simulink library "acc"  (R2021b)
settings: Solver=VariableStepAuto  StartTime=0.0  StopTime=10.0  RelTol=1e-3
undefined symbols (not defined in the file or in its folder): AACC_CondensorFanReq_X_enum, AACC_EWP1CCUReq_X_C, AACC_EWP1EDUReq_X_C, AACC_EWP1HVBReq_X_C, AACC_EWP2CCUReq_X_C, AACC_EWP2EDUReq_X_C, AACC_EWP2HVBReq_X_C, AACC_FWV1CCUReq_X_C, AACC_FWV1EDUReq_X_C, AACC_FWV1HVBReq_X_C, AACC_FWV2CCUReq_X_C, AACC_FWV2EDUReq_X_C, AACC_FWV2HVBReq_X_C, AACC_TWVCCUReq_X_C, AACC_TWVEDUReq_X_C, AACC_TWVHVBReq_X_C, ENUM_ACCMODE_CHARGING, ENUM_ACCMODE_COOLING, ENUM_ACCMODE_OFF, ENUM_ACCMODE_SERVICE, ENUM_ACREQ_COOLING, ENUM_ACREQ_NOREQUEST, ENUM_CHILLERINITREQ_NONE, ENUM_CHILLERINITREQ_START, ENUM_CHILLERINITREQ_WAITING, ENUM_CHILLERINITSTA_FINISH, ENUM_CHILLERINITSTA_INPROCESS, ENUM_COOLFANREQ_HI, ENUM_COOLFANREQ_LOW, ENUM_COOLFANREQ_OFF, ENUM_LVBATTSTA_FAIL, ENUM_LVBATTSTA_NORMAL, ENUM_PMMMODE_CHARGE, ENUM_PMMMODE_DRIVE, ENUM_PMMMODE_LVBATCHRG, ENUM_PMMMODE_POWERUP, ENUM_THCMSYS_INACTIVE, FALSE, KACC_CCUFanHighOffTemp_C, KACC_CCUFanHighOnTemp_C, KACC_CCUFanLowOffTemp_C, KACC_CCUFanLowOnTemp_C, KACC_ChillerInitTime_s, KACC_ChillerStartTime_s, KACC_DCDCCalPwrAvailRsv_kW, KACC_EDUFanHighOffTemp_C, KACC_EDUFanHighOnTemp_C, KACC_EDUFanLowOffTemp_C, KACC_EDUFanLowOnTemp_C, KACC_EWP1CalDutyVal_pct, KACC_EWP1CalON_flg, KACC_EWP2CalDutyVal_pct, KACC_EWP2CalON_flg, KACC_EXVCalON_flg, KACC_EXVCalVal_cnt, KACC_FanCalON_flg, KACC_FanCalVal_enum, KACC_FWV1CalON_flg, KACC_FWV1CalVal_flg, KACC_FWV2CalON_flg ... (+51)
libraries: simulink x1
(part 2 of 2)

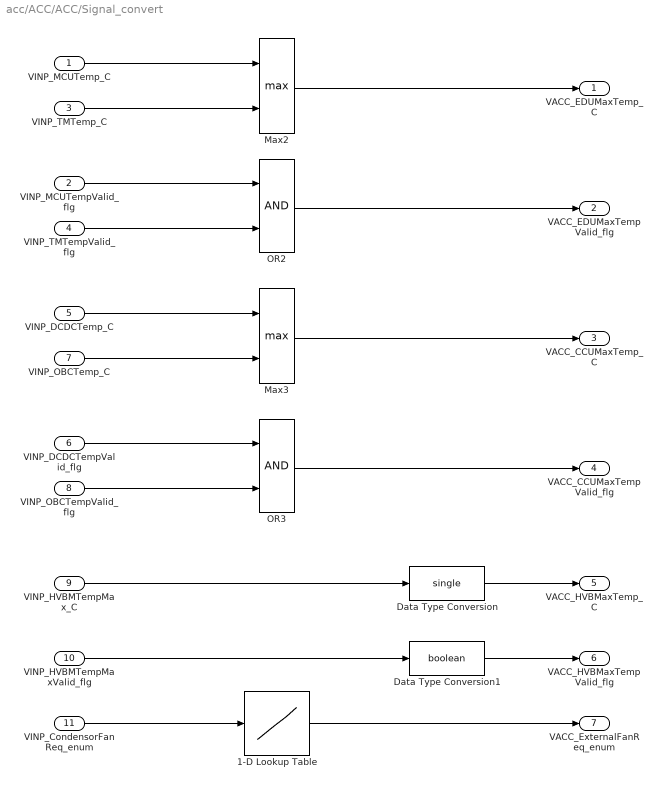
== system acc/ACC/ACC/Signal_convert ==
  VINP_MCUTemp_C : Inport
  VINP_MCUTempValid_flg : Inport  Port=2
  VINP_TMTemp_C : Inport  Port=3
  VINP_TMTempValid_flg : Inport  Port=4
  VINP_DCDCTemp_C : Inport  Port=5
  VINP_DCDCTempValid_flg : Inport  Port=6
  VINP_OBCTemp_C : Inport  Port=7
  VINP_OBCTempValid_flg : Inport  Port=8
  VINP_HVBMTempMax_C : Inport  Port=9
  VINP_HVBMTempMaxValid_flg : Inport  Port=10
  VINP_CondensorFanReq_enum : Inport  Port=11
  1-D Lookup Table : Lookup_n-D  NumberOfTableDimensions=1  BreakpointsForDimension1=AACC_CondensorFanReq_X_enum  Table=MACC_CondensorFanReq_Y_enum  InterpMethod=Flat  InternalRulePriority=Speed  RndMeth=Simplest  InputSameDT=on
  Data Type Conversion : DataTypeConversion  OutDataTypeStr=single
  Data Type Conversion1 : DataTypeConversion  OutDataTypeStr=boolean
  Max2 : MinMax  Function=max  Inputs=2
  Max3 : MinMax  Function=max  Inputs=2
  OR2 : Logic  AllPortsSameDT=off  OutDataTypeStr=boolean
  OR3 : Logic  AllPortsSameDT=off  OutDataTypeStr=boolean
  VACC_EDUMaxTemp_C : Outport
  VACC_EDUMaxTempValid_flg : Outport  Port=2
  VACC_CCUMaxTemp_C : Outport  Port=3
  VACC_CCUMaxTempValid_flg : Outport  Port=4
  VACC_HVBMaxTemp_C : Outport  Port=5
  VACC_HVBMaxTempValid_flg : Outport  Port=6
  VACC_ExternalFanReq_enum : Outport  Port=7
  wires:
  Data Type Conversion1/1 -> VACC_HVBMaxTempValid_flg/1
  Data Type Conversion/1 -> VACC_HVBMaxTemp_C/1
  1-D Lookup Table/1 -> VACC_ExternalFanReq_enum/1
  VINP_CondensorFanReq_enum/1 -> 1-D Lookup Table/1
  VINP_HVBMTempMaxValid_flg/1 -> Data Type Conversion1/1
  VINP_HVBMTempMax_C/1 -> Data Type Conversion/1
  OR3/1 -> VACC_CCUMaxTempValid_flg/1
  Max3/1 -> VACC_CCUMaxTemp_C/1
  VINP_OBCTempValid_flg/1 -> OR3/2
  VINP_DCDCTempValid_flg/1 -> OR3/1
  VINP_DCDCTemp_C/1 -> Max3/1
  VINP_OBCTemp_C/1 -> Max3/2
  OR2/1 -> VACC_EDUMaxTempValid_flg/1
  VINP_TMTempValid_flg/1 -> OR2/2
  VINP_MCUTempValid_flg/1 -> OR2/1
  Max2/1 -> VACC_EDUMaxTemp_C/1
  VINP_TMTemp_C/1 -> Max2/2
  VINP_MCUTemp_C/1 -> Max2/1

== system acc/ACC/ACC/Thermal_Managemant_Mode_Determination ==
  VPMM_SysPowerMode_enum : Inport
  Constant : Constant  Value=KACC_ServiceModeON_flg
  Cooling Mode : Subsystem
  PECoolingMode : Subsystem
  Service Mode : Subsystem
  Subsystem : Subsystem
  VACC_PECoolingMode_enum : Outport  VectorParamsAs1DForOutWhenUnconnected=off
  wires:
  Constant/1 -> Service Mode/1(KACC_ServiceModeON_flg)
  [VACC_CoolingMode_flg] -> PECoolingMode/3(VACC_CoolingMode_flg)
  [VACC_ChargingMode_flg] -> PECoolingMode/2(VACC_ChargingMode_flg)
  [VACC_ServiceMode_flg] -> PECoolingMode/1(VACC_ServiceMode_flg)
  [VPMM_SysPowerMode_enum] -> Subsystem/1(VPMM_SysPowerMode_enum)
  Subsystem/1(VACC_CoolingMode_flg) -> [VACC_CoolingMode_flg]
  PECoolingMode/1(VACC_PECoolingMode_enum) -> VACC_PECoolingMode_enum/1
  [VPMM_SysPowerMode_enum] -> Cooling Mode/1(VPMM_SysPowerMode_enum)
  VPMM_SysPowerMode_enum/1 -> [VPMM_SysPowerMode_enum]
  Service Mode/1(VACC_ServiceMode_flg) -> [VACC_ServiceMode_flg]
  Cooling Mode/1(VACC_ChargingMode_flg) -> [VACC_ChargingMode_flg]

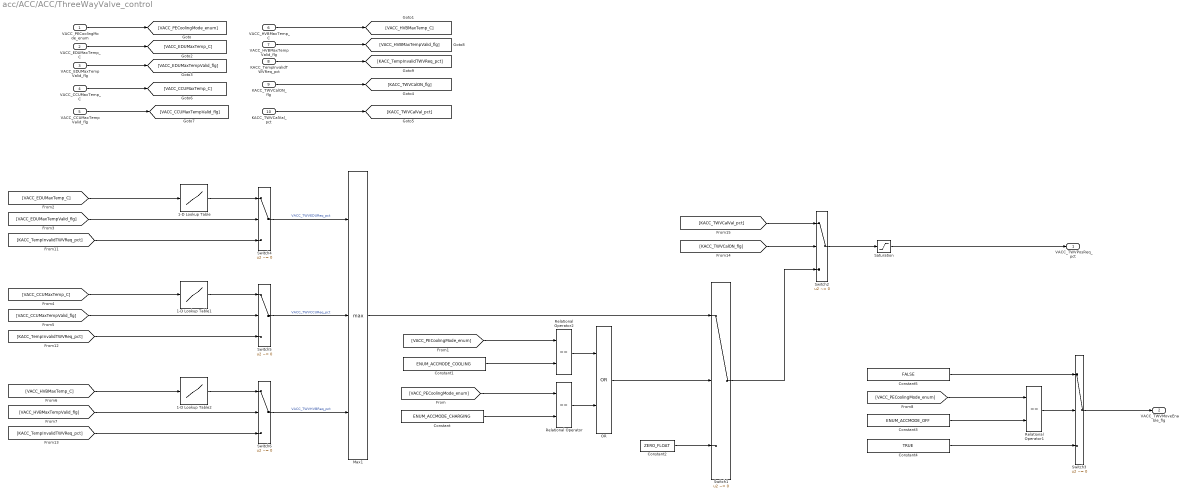
== system acc/ACC/ACC/ThreeWayValve_control ==
  VACC_PECoolingMode_enum : Inport
  VACC_EDUMaxTemp_C : Inport  Port=2
  VACC_EDUMaxTempValid_flg : Inport  Port=3
  VACC_CCUMaxTemp_C : Inport  Port=4
  VACC_CCUMaxTempValid_flg : Inport  Port=5
  VACC_HVBMaxTemp_C : Inport  Port=6
  VACC_HVBMaxTempValid_flg : Inport  Port=7
  KACC_TempInvalidTWVReq_pct : Inport  Port=8
  KACC_TWVCalON_flg : Inport  Port=9
  KACC_TWVCalVal_pct : Inport  Port=10
  1-D Lookup Table : Lookup_n-D  NumberOfTableDimensions=1  BreakpointsForDimension1=AACC_TWVEDUReq_X_C  Table=MACC_TWVEDUReq_Y_pct  UseLastTableValue=on  InternalRulePriority=Speed  RndMeth=Simplest  InputSameDT=on
  1-D Lookup Table1 : Lookup_n-D  NumberOfTableDimensions=1  BreakpointsForDimension1=AACC_TWVCCUReq_X_C  Table=MACC_TWVCCUReq_Y_pct  UseLastTableValue=on  InternalRulePriority=Speed  RndMeth=Simplest  InputSameDT=on
  1-D Lookup Table2 : Lookup_n-D  NumberOfTableDimensions=1  BreakpointsForDimension1=AACC_TWVHVBReq_X_C  Table=MACC_TWVHVBReq_Y_pct  UseLastTableValue=on  InternalRulePriority=Speed  RndMeth=Simplest  InputSameDT=on
  Constant : Constant  Value=ENUM_ACCMODE_CHARGING
  Constant1 : Constant  Value=ENUM_ACCMODE_COOLING
  Constant2 : Constant  Value=ZERO_FLOAT
  Constant3 : Constant  Value=ENUM_ACCMODE_OFF
  Constant4 : Constant  Value=TRUE
  Constant5 : Constant  Value=FALSE
  Max1 : MinMax  Function=max  Inputs=3
  OR : Logic  Operator=OR  AllPortsSameDT=off  OutDataTypeStr=boolean
  Relational Operator : RelationalOperator  Operator===  OutDataTypeStr=boolean  RndMeth=Simplest
  Relational Operator1 : RelationalOperator  Operator===  OutDataTypeStr=boolean  RndMeth=Simplest
  Relational Operator2 : RelationalOperator  Operator===  OutDataTypeStr=boolean  RndMeth=Simplest
  Saturation : Saturate  UpperLimit=100  LowerLimit=0
      settings: AttributesFormatString=|
      | LowerLimi: %<LowerLimit>
      | UpperLimit: %<UpperLimit>
  Switch{1..6} (6 alike) : Switch  Criteria=u2 ~= 0
      settings: AttributesFormatString=%<Criteria>
  VACC_TWVPosReq_pct : Outport
  VACC_TWVMoveEnable_flg : Outport  Port=2
  wires:
  Constant4/1 -> Switch3/3
  Constant5/1 -> Switch3/1
  Switch3/1 -> VACC_TWVMoveEnable_flg/1
  Relational Operator1/1 -> Switch3/2
  [VACC_PECoolingMode_enum] -> Relational Operator1/1
  Constant3/1 -> Relational Operator1/2
  Switch5/1 -> Max1/2  "VACC_TWVCCUReq_pct"
  Switch4/1 -> Max1/1  "VACC_TWVEDUReq_pct"
  KACC_TempInvalidTWVReq_pct/1 -> [KACC_TempInvalidTWVReq_pct]
  VACC_HVBMaxTempValid_flg/1 -> [VACC_HVBMaxTempValid_flg]
  VACC_CCUMaxTempValid_flg/1 -> [VACC_CCUMaxTempValid_flg]
  VACC_CCUMaxTemp_C/1 -> [VACC_CCUMaxTemp_C]
  VACC_EDUMaxTempValid_flg/1 -> [VACC_EDUMaxTempValid_flg]
  VACC_EDUMaxTemp_C/1 -> [VACC_EDUMaxTemp_C]
  Constant2/1 -> Switch1/3
  OR/1 -> Switch1/2
  Relational Operator/1 -> OR/2
  Relational Operator2/1 -> OR/1
  VACC_HVBMaxTemp_C/1 -> [VACC_HVBMaxTemp_C]
  Switch1/1 -> Switch2/3
  Constant/1 -> Relational Operator/2
  Constant1/1 -> Relational Operator2/2
  Max1/1 -> Switch1/1
  [VACC_PECoolingMode_enum] -> Relational Operator2/1
  [VACC_PECoolingMode_enum] -> Relational Operator/1
  VACC_PECoolingMode_enum/1 -> [VACC_PECoolingMode_enum]
  Switch2/1 -> Saturation/1
  Saturation/1 -> VACC_TWVPosReq_pct/1
  KACC_TWVCalON_flg/1 -> [KACC_TWVCalON_flg]
  KACC_TWVCalVal_pct/1 -> [KACC_TWVCalVal_pct]
  [VACC_EDUMaxTempValid_flg] -> Switch4/2
  [KACC_TempInvalidTWVReq_pct] -> Switch4/3
  [VACC_EDUMaxTemp_C] -> 1-D Lookup Table/1
  1-D Lookup Table/1 -> Switch4/1
  [VACC_CCUMaxTemp_C] -> 1-D Lookup Table1/1
  1-D Lookup Table1/1 -> Switch5/1
  [VACC_CCUMaxTempValid_flg] -> Switch5/2
  [KACC_TempInvalidTWVReq_pct] -> Switch5/3
  Switch6/1 -> Max1/3  "VACC_TWVHVBReq_pct"
  1-D Lookup Table2/1 -> Switch6/1
  [VACC_HVBMaxTempValid_flg] -> Switch6/2
  [VACC_HVBMaxTemp_C] -> 1-D Lookup Table2/1
  [KACC_TempInvalidTWVReq_pct] -> Switch6/3
  [KACC_TWVCalON_flg] -> Switch2/2
  [KACC_TWVCalVal_pct] -> Switch2/1

== system acc/ACC/THCM/THCM_Available_Check ==
  VPMM_HVPwrSta_flg : Inport
  Constant4 : Constant  Value=ENUM_THCMSYS_INACTIVE
  Constant5 : Constant  Value=KACC_HVTHCMSysAvail_enum_ovrdflg
  Constant6 : Constant  Value=KACC_HVTHCMSysAvail_enum_ovrdval
  Constant7 : Constant  Value=ENUM_THCMSYS_INACTIVE
  Switch2 : Switch  Criteria=u2 ~= 0
      settings: AttributesFormatString=<%<Criteria>>
  Switch3 : Switch  Criteria=u2 ~= 0
      settings: AttributesFormatString=<%<Criteria>>
  VACC_HVTHCMSysAvail_enum : Outport
  wires:
  Constant5/1 -> Switch3/2
  Constant4/1 -> Switch2/3
  Switch2/1 -> VACC_HVTHCMSysAvail_enum/1  "VACC_HVTHCMSysAvail_enum"
  Switch3/1 -> Switch2/1
  VPMM_HVPwrSta_flg/1 -> Switch2/2
  Constant6/1 -> Switch3/1
  Constant7/1 -> Switch3/3

== system acc/ACC/THCM/THCM_Available_Power ==
  VPMM_HVPwrSta_flg : Inport
  VINP_HVBPwrAvailDchrg_kW : Inport  Port=2
  VINP_FrMCUDCBusVolt_V : Inport  Port=3
  VINP_FrMCUDCBusCurr_A : Inport  Port=4
  VINP_RrMCUDCBusVolt_V : Inport  Port=5
  VINP_RrMCUDCBusCurr_A : Inport  Port=6
  Add : Sum
  Add1 : Sum  Inputs=+-
  Constant10 : Constant  Value=KACC_HVPwrAvail4THCM_W_ovrdval
  Constant8 : Constant  Value=ZERO_FLOAT
  Constant9 : Constant  Value=KACC_HVPwrAvail4THCM_W_ovrdflg
  Product : Product
  Product1 : Product
  Saturation : Saturate  UpperLimit=KACC_THCMMaxPwrAvail_W  LowerLimit=0
      settings: AttributesFormatString=|
      | Upper Limit: %<UpperLimit>
      | Lower Limit: %<LowerLimit>
  Switch1 : Switch  Criteria=u2 ~= 0
      settings: AttributesFormatString=<%<Criteria>>
  Switch4 : Switch  Criteria=u2 ~= 0
      settings: AttributesFormatString=<%<Criteria>>
  VACC_VehHVPwrAvail4THCM_W : Outport
  wires:
  Constant10/1 -> Switch4/1
  Switch4/1 -> Switch1/1
  Saturation/1 -> Switch4/3
  Constant8/1 -> Switch1/3
  VPMM_HVPwrSta_flg/1 -> Switch1/2
  Switch1/1 -> VACC_VehHVPwrAvail4THCM_W/1  "VACC_VehHVPwrAvail4THCM_W"
  Constant9/1 -> Switch4/2
  VINP_RrMCUDCBusCurr_A/1 -> Product/2
  VINP_RrMCUDCBusVolt_V/1 -> Product/1
  VINP_FrMCUDCBusCurr_A/1 -> Product1/2
  VINP_FrMCUDCBusVolt_V/1 -> Product1/1
  Product1/1 -> Add/1
  Product/1 -> Add/2
  VINP_HVBPwrAvailDchrg_kW/1 -> Add1/1
  Add/1 -> Add1/2
  Add1/1 -> Saturation/1

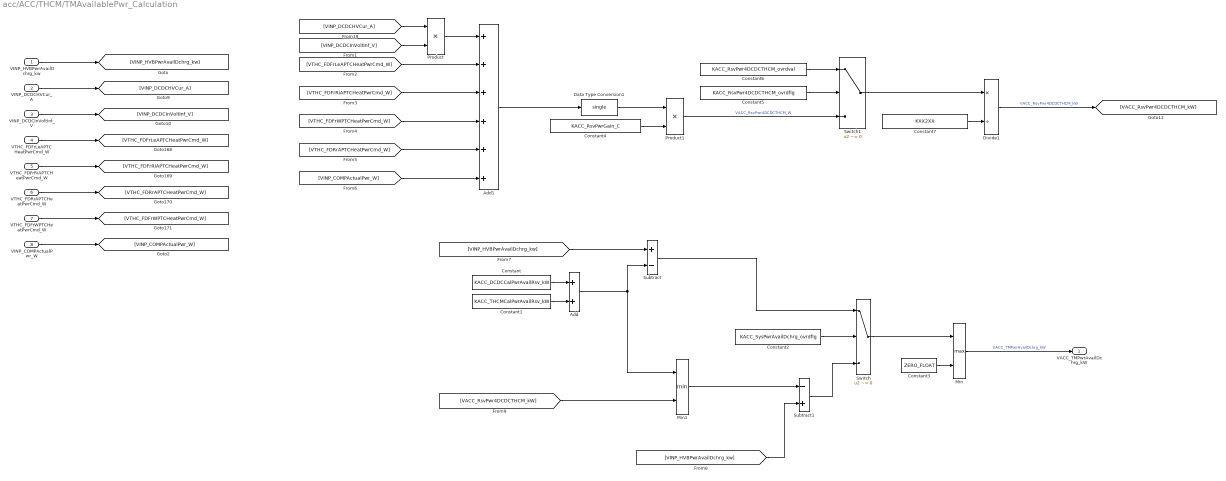
== system acc/ACC/THCM/TMAvailablePwr_Calculation ==
  VINP_HVBPwrAvailDchrg_kw : Inport
  VINP_DCDCHVCur_A : Inport  Port=2
  VINP_DCDCInVoltInf_V : Inport  Port=3
  VTHC_FDFrLeAPTCHeatPwrCmd_W : Inport  Port=4
  VTHC_FDFrRiAPTCHeatPwrCmd_W : Inport  Port=5
  VTHC_FDRrAPTCHeatPwrCmd_W : Inport  Port=6
  VTHC_FDFrWPTCHeatPwrCmd_W : Inport  Port=7
  VINP_COMPActualPwr_W : Inport  Port=8
  Add : Sum
  Add1 : Sum  Inputs=++++++
  Constant : Constant  Value=KACC_DCDCCalPwrAvailRsv_kW
  Constant1 : Constant  Value=KACC_THCMCalPwrAvailRsv_kW
  Constant2 : Constant  Value=KACC_SysPwrAvailDchrg_ovrdflg
  Constant3 : Constant  Value=ZERO_FLOAT
  Constant4 : Constant  Value=KACC_RsvPwrGain_C
  Constant5 : Constant  Value=KACC_RsvPwr4DCDCTHCM_ovrdflg
  Constant6 : Constant  Value=KACC_RsvPwr4DCDCTHCM_ovrdval
  Constant7 : Constant  Value=KXX2XX
  Data Type Conversion1 : DataTypeConversion  OutDataTypeStr=single
  Divide1 : Product  Inputs=*/
  Min : MinMax  Function=max  Inputs=2
  Min1 : MinMax  Inputs=2
  Product : Product
  Product1 : Product
  Subtract : Sum  Inputs=+-
  Subtract1 : Sum  Inputs=-+
  Switch : Switch  Criteria=u2 ~= 0
      settings: AttributesFormatString=<%<Criteria>>
  Switch1 : Switch  Criteria=u2 ~= 0
  VACC_TMPwrAvailDchrg_kW : Outport
  wires:
  Min1/1 -> Subtract1/1
  [VINP_HVBPwrAvailDchrg_kw] -> Subtract1/2
  [VINP_HVBPwrAvailDchrg_kw] -> Subtract/1
  Subtract1/1 -> Switch/3
  [VACC_RsvPwr4DCDCTHCM_kW] -> Min1/2
  Data Type Conversion1/1 -> Product1/1
  Constant5/1 -> Switch1/2
  Add1/1 -> Data Type Conversion1/1
  Switch1/1 -> Divide1/1
  Divide1/1 -> [VACC_RsvPwr4DCDCTHCM_kW]  "VACC_RsvPwr4DCDCTHCM_kW"
  [VINP_DCDCInVoltInf_V] -> Product/2
  [VINP_DCDCHVCur_A] -> Product/1
  Product/1 -> Add1/1
  [VTHC_FDRrAPTCHeatPwrCmd_W] -> Add1/5
  Constant6/1 -> Switch1/1
  Constant4/1 -> Product1/2
  [VTHC_FDFrRiAPTCHeatPwrCmd_W] -> Add1/3
  Product1/1 -> Switch1/3  "VACC_RsvPwr4DCDCTHCM_W"
  [VINP_COMPActualPwr_W] -> Add1/6
  [VTHC_FDFrLeAPTCHeatPwrCmd_W] -> Add1/2
  [VTHC_FDFrWPTCHeatPwrCmd_W] -> Add1/4
  Constant7/1 -> Divide1/2
  VINP_COMPActualPwr_W/1 -> [VINP_COMPActualPwr_W]
  VTHC_FDFrWPTCHeatPwrCmd_W/1 -> [VTHC_FDFrWPTCHeatPwrCmd_W]
  VTHC_FDRrAPTCHeatPwrCmd_W/1 -> [VTHC_FDRrAPTCHeatPwrCmd_W]
  VTHC_FDFrRiAPTCHeatPwrCmd_W/1 -> [VTHC_FDFrRiAPTCHeatPwrCmd_W]
  VTHC_FDFrLeAPTCHeatPwrCmd_W/1 -> [VTHC_FDFrLeAPTCHeatPwrCmd_W]
  VINP_DCDCInVoltInf_V/1 -> [VINP_DCDCInVoltInf_V]
  VINP_DCDCHVCur_A/1 -> [VINP_DCDCHVCur_A]
  Constant/1 -> Add/1
  Constant1/1 -> Add/2
  VINP_HVBPwrAvailDchrg_kw/1 -> [VINP_HVBPwrAvailDchrg_kw]
  Add/1 -> Subtract/2, Min1/1
  Subtract/1 -> Switch/1
  Constant2/1 -> Switch/2
  Switch/1 -> Min/1
  Min/1 -> VACC_TMPwrAvailDchrg_kW/1  "VACC_TMPwrAvailDchrg_kW"
  Constant3/1 -> Min/2

== system acc/ACC/ACC/Thermal_Managemant_Mode_Determination/Cooling Mode ==
  VPMM_SysPowerMode_enum : Inport
  Constant2 : Constant  Value=ENUM_PMMMODE_LVBATCHRG  SampleTime=-1
  Constant4 : Constant  Value=ENUM_PMMMODE_CHARGE  SampleTime=-1
  Logical Operator : Logic  Operator=OR  AllPortsSameDT=off  OutDataTypeStr=boolean
  Relational Operator1 : RelationalOperator  Operator===  OutDataTypeStr=boolean  RndMeth=Nearest
  Relational Operator3 : RelationalOperator  Operator===  OutDataTypeStr=boolean  RndMeth=Nearest
  VACC_ChargingMode_flg : Outport  VectorParamsAs1DForOutWhenUnconnected=off
  wires:
  [VPMM_SysPowerMode_enum] -> Relational Operator3/1
  Constant2/1 -> Relational Operator3/2
  VPMM_SysPowerMode_enum/1 -> [VPMM_SysPowerMode_enum]
  [VPMM_SysPowerMode_enum] -> Relational Operator1/1
  Constant4/1 -> Relational Operator1/2
  Relational Operator3/1 -> Logical Operator/1
  Relational Operator1/1 -> Logical Operator/2
  Logical Operator/1 -> VACC_ChargingMode_flg/1  "VACC_ChargingMode_flg"

== system acc/ACC/ACC/Thermal_Managemant_Mode_Determination/PECoolingMode ==
  VACC_ServiceMode_flg : Inport
  VACC_ChargingMode_flg : Inport  Port=2
  VACC_CoolingMode_flg : Inport  Port=3
  Constant12 : Constant  Value=ENUM_ACCMODE_COOLING  SampleTime=-1
  Constant15 : Constant  Value=ENUM_ACCMODE_OFF  SampleTime=-1
  Constant2 : Constant  Value=ENUM_ACCMODE_CHARGING  SampleTime=-1
  Constant7 : Constant  Value=ENUM_ACCMODE_SERVICE  SampleTime=-1
  Switch1 : Switch  Criteria=u2 ~= 0
  Switch2 : Switch  Criteria=u2 ~= 0
  Switch4 : Switch  Criteria=u2 ~= 0
  VACC_PECoolingMode_enum : Outport  VectorParamsAs1DForOutWhenUnconnected=off
  wires:
  Constant15/1 -> Switch1/3
  Switch4/1 -> VACC_PECoolingMode_enum/1  "VACC_PECoolingMode_enum"
  VACC_CoolingMode_flg/1 -> Switch1/2
  Constant12/1 -> Switch1/1
  VACC_ServiceMode_flg/1 -> Switch4/2
  Constant7/1 -> Switch4/1
  Switch2/1 -> Switch4/3
  VACC_ChargingMode_flg/1 -> Switch2/2
  Switch1/1 -> Switch2/3
  Constant2/1 -> Switch2/1

== system acc/ACC/ACC/Thermal_Managemant_Mode_Determination/Service Mode ==
  KACC_ServiceModeON_flg : Inport
  VACC_ServiceMode_flg : Outport  VectorParamsAs1DForOutWhenUnconnected=off
  wires:
  KACC_ServiceModeON_flg/1 -> VACC_ServiceMode_flg/1  "VACC_ServiceMode_flg"

== system acc/ACC/ACC/Thermal_Managemant_Mode_Determination/Subsystem ==
  VPMM_SysPowerMode_enum : Inport
  Constant1 : Constant  Value=ENUM_PMMMODE_DRIVE  SampleTime=-1
  Constant2 : Constant  Value=ENUM_PMMMODE_POWERUP  SampleTime=-1
  Logical Operator : Logic  Operator=OR  AllPortsSameDT=off  OutDataTypeStr=boolean
  Relational Operator1 : RelationalOperator  Operator===  OutDataTypeStr=boolean  RndMeth=Nearest
  Relational Operator2 : RelationalOperator  Operator===  OutDataTypeStr=boolean  RndMeth=Nearest
  VACC_CoolingMode_flg : Outport  VectorParamsAs1DForOutWhenUnconnected=off
  wires:
  Logical Operator/1 -> VACC_CoolingMode_flg/1  "VACC_CoolingMode_flg"
  Relational Operator1/1 -> Logical Operator/2
  Relational Operator2/1 -> Logical Operator/1
  VPMM_SysPowerMode_enum/1 -> [VPMM_SysPowerMode_enum]
  [VPMM_SysPowerMode_enum] -> Relational Operator2/1
  [VPMM_SysPowerMode_enum] -> Relational Operator1/1
  Constant1/1 -> Relational Operator1/2
  Constant2/1 -> Relational Operator2/2

== stateflow chart acc/ACC/THCM/LVBattSta_Check ==
  state Check_LV_Batt
    state Check_LVBatt_Low
      en:
      VACC_ChkLVBattLowPass_flg = FALSE;
      (default) -> (junction 148) : {VACC_LVBattChkTime_s = 0;}
      (junction 148) -> (junction 149) [order 1] : [VINP_LVBattDet12V_V > KACC_LVBattErrLoThd_V]
      Check_LVBatt_Low -> (junction 148) [order 1]
      (junction 148) -> (junction 150) [order 2] : {VACC_LVBattChkTime_s += task_time_s;}
      (junction 149) -> (junction 151) : {VACC_ChkLVBattLowPass_flg = TRUE;}
      (junction 151) -> (junction 150)
    state Check_LVBatt_High
      en:
      VACC_ChkLVBattHighPass_flg = FALSE;
      (default) -> (junction 159) : {VACC_LVBattChkTime_s = 0;}
      Check_LVBatt_High -> (junction 159) [order 1]
      (junction 159) -> (junction 160) [order 1] : [VINP_LVBattDet12V_V < KACC_LVBattErrHiThd_V]
      (junction 159) -> (junction 161) [order 2] : {VACC_LVBattChkTime_s += task_time_s;}
      (junction 160) -> (junction 162) : {VACC_ChkLVBattHighPass_flg = TRUE;}
      (junction 162) -> (junction 161)
    state Check_LVBatt_Pass
      en:
      VACC_LVBattVoltSta_enum = ENUM_LVBATTSTA_NORMAL;
    state Check_LVBatt_Fail
      en:
      VACC_LVBattVoltSta_enum = ENUM_LVBATTSTA_FAIL;
    (default) -> (junction 130)
    (junction 182) -> (junction 130)
    (junction 180) -> (junction 182)
    (junction 130) -> (junction 132)
    (junction 132) -> (junction 131) [order 2]
    (junction 131) -> Check_LVBatt_Pass
    (junction 132) -> Check_LVBatt_Low [order 1] : [VPMM_LVPwrSta_flg]
    Check_LVBatt_Low -> (junction 133) [order 2] : [VACC_LVBattChkTime_s > KACC_LVBattErrFailtime_s]
    (junction 133) -> (junction 134)
    Check_LVBatt_Low -> Check_LVBatt_High [order 1] : [VACC_ChkLVBattLowPass_flg]
    Check_LVBatt_High -> (junction 134) [order 2] : [VACC_LVBattChkTime_s > KACC_LVBattErrFailtime_s]
    (junction 134) -> Check_LVBatt_Fail
    Check_LVBatt_High -> Check_LVBatt_Pass [order 1] : [VACC_ChkLVBattHighPass_flg]
    Check_LVBatt_Pass -> (junction 173)
    Check_LVBatt_Fail -> (junction 175)
    (junction 173) -> (junction 180)
    (junction 175) -> (junction 173)
  data: task_time_s input; VPMM_LVPwrSta_flg input; VINP_LVBattDet12V_V input; KACC_LVBattErrLoThd_V input; KACC_LVBattErrHiThd_V input; KACC_LVBattErrFailtime_s input; VACC_LVBattVoltSta_enum output uint8; VACC_ChkLVBattHighPass_flg local boolean; VACC_ChkLVBattLowPass_flg local boolean; VACC_LVBattChkTime_s local single; ENUM_LVBATTSTA_FAIL parameter; ENUM_LVBATTSTA_NORMAL parameter; FALSE parameter; TRUE parameter

== stateflow chart acc/ACC/ACC/Chiller_control/Chiller_Initialize ==
  state MainInitialize
    en:
    VACC_ChillerInitFinish_flg = FALSE;
    VACC_ChillerInitTimeout_flg = FALSE;
    VACC_ChillerInitStart_flg = FALSE;
    VACC_ChillerInitReq_enum = ENUM_CHILLERINITREQ_NONE;
    VACC_ChillerMoveEnable_flg = FALSE;
  state ChillerInitialize
    (default) -> (junction 10) : {
        | VACC_TimeChillerInit_s = 0;
        | }
    ChillerInitialize -> (junction 10) [order 1]
    (junction 10) -> (junction 11) : {
        | VACC_ChillerInitReq_enum = ENUM_CHILLERINITREQ_START;
        | VACC_ChillerMoveEnable_flg = TRUE;
        | }
    (junction 11) -> (junction 13) [order 1] : [VINP_ChillerInitState_enum == ENUM_CHILLERINITSTA_INPROCESS]
    (junction 11) -> (junction 17) [order 2] : {
        | VACC_TimeChillerInit_s  += task_time_s;
        | }
    (junction 13) -> (junction 15) : {
        | VACC_ChillerInitStart_flg = TRUE;
        | }
    (junction 15) -> (junction 17)
  state Timeout
    en:
    VACC_ChillerInitTimeout_flg = TRUE;
    VACC_ChillerMoveEnable_flg = FALSE;
  state ChillerStart
    (default) -> (junction 28) : {
        | VACC_TimeChillerStart_s = 0;
        | }
    ChillerStart -> (junction 28) [order 1]
    (junction 28) -> (junction 29) : {
        | VACC_ChillerInitReq_enum = ENUM_CHILLERINITREQ_WAITING;
        | }
    (junction 29) -> (junction 30) [order 1] : [VINP_ChillerInitState_enum == ENUM_CHILLERINITSTA_FINISH]
    (junction 29) -> (junction 31) [order 2] : {
        | VACC_TimeChillerStart_s += task_time_s;
        | }
    (junction 30) -> (junction 32) : {
        | VACC_ChillerInitFinish_flg = TRUE;
        | VACC_ChillerInitReq_enum = ENUM_CHILLERINITREQ_NONE;
        | }
    (junction 32) -> (junction 31)
  (default) -> MainInitialize
  MainInitialize -> ChillerInitialize : [VACC_PECoolingMode_enum == ENUM_ACCMODE_COOLING ||...
      | VACC_PECoolingMode_enum == ENUM_ACCMODE_CHARGING]
  ChillerInitialize -> Timeout [order 2] : [VACC_TimeChillerInit_s > KACC_ChillerInitTime_s]
  ChillerInitialize -> ChillerStart [order 1] : [VACC_ChillerInitStart_flg]
  ChillerStart -> Timeout [order 1] : [VACC_TimeChillerStart_s > KACC_ChillerStartTime_s]
  data: KACC_ChillerInitTime_s input; KACC_ChillerStartTime_s input; VACC_PECoolingMode_enum input; VINP_ChillerInitState_enum input; task_time_s input; VACC_ChillerInitFinish_flg output; VACC_ChillerInitReq_enum output; VACC_ChillerInitTimeout_flg output; VACC_ChillerInitStart_flg local boolean; VACC_TimeChillerInit_s local single; ENUM_ACCMODE_CHARGING parameter; ENUM_ACCMODE_COOLING parameter; ENUM_CHILLERINITREQ_NONE parameter; ENUM_CHILLERINITREQ_START parameter; ENUM_CHILLERINITSTA_FINISH parameter; ENUM_CHILLERINITSTA_INPROCESS parameter; FALSE parameter; TRUE parameter; VACC_TimeChillerStart_s local single; ENUM_CHILLERINITREQ_WAITING parameter; VACC_ChillerMoveEnable_flg output boolean
